simulink model "positionControlSlidingCircle"  (Simulink 7.5)
settings: Solver=FixedStepDiscrete  StartTime=0.0  StopTime=Inf  FixedStep=Ts  RelTol=1e-3
PostLoadFcn:
  | , if any(exist('dsrtsu_mdlpostloadfcn', 'file') == [2, 3, 6]), try dsrtsu_mdlpostloadfcn('Execute', bdroot); catch fprintf('Error in PostLoadFcn (dsrtsu_mdlpostloadfcn) for model "%s":\n %s\n', bdroot, lasterr); end, end,
values from neighbouring files (symbols this model uses):
  bLP = exp(-Wcut*2*pi*Ts)    [main2.m]
  circX = circXt(1:floor(length(circXt)))    [main.m]    (also in main2.m = circX(1:floor(length(circX)/factor)))
  circXd = circXd(1:floor(length(circX)/factor))    [main2.m]
  circXdd = circXdd(1:floor(length(circX)/factor))    [main2.m]
  circY = circYt(1:floor(length(circYt)))    [main.m]    (also in main2.m = circY(1:floor(length(circY)/factor)))
  circYd = circYd(1:floor(length(circY)/factor))    [main2.m]
  circYdd = circYdd(1:floor(length(circY)/factor))    [main2.m]
  cx = 0.001651705312519    (= 0.00165170531252)    [main2.m]
  cy = 0.001046707328795    (= 0.00104670732879)    [main2.m]
  Kd = [5 0;0 5]*10^-4    [main2.m]
  kNorm = 1*10^-1    (= 0.1)    [main2.m]
  Kp = [8 0; 0 7]*10^-2    [main2.m]
  Ks = [7 0;0 0.7]*10^-2    [main2.m]
  Minv = inv(M)    [main2.m]
  mx = 9.241410334340282e-004    (= 0.000924141033434)    [main2.m]
  my = 5.572114462326005e-004    (= 0.000557211446233)    [main2.m]
  r0 = rad    [main2.m]
  rNormal = 109.08    [main2.m]
  Ts = 0.01    [main.m]    (also in main2.m = 0.001)
undefined symbols (not defined in the file or in its folder): DiscIntNeverNeededParam, xc, yc
libraries: rtilib1103 x12, dspinverses x2, dspmtrx3 x2
settings Model: DSRTSU_INTERNAL_RTI_VER=360  DSRTSU_INTERNAL_RTI_TYPE=rti1103  Creator=daq  LastModifiedBy=daq  BufferReuse=off
settings OptimizationCC: BlockReduction=off  OptimizeBlockIOStorage=off  BufferReuse=off  ExpressionFolding=off  LocalBlockOutputs=off
settings HardwareCC: ProdIntDivRoundTo=Zero  ProdEndianess=BigEndian  ProdHWDeviceType=Generic->Custom  TargetIntDivRoundTo=Zero  TargetEndianess=BigEndian  TargetHWDeviceType=Generic->Custom
settings RTWCC: SystemTargetFile=rti1103.tlc  MakeCommand=make_rti  TemplateMakefile=rti1103.tmf  Description=dSPACE DS1103 Hardware Platform  ProcessScript=rti1103_make_rtw_hook
settings STFCustomTargetCC: ParMdlRefBuildCompliant=on  GeneratePreprocessorConditionals=Disable all  SystemTargetFile=rti1103.tlc
settings GRTTargetCC: CompOptLevelCompliant=off  MatFileLogging=off  ExtModeMexFile=noextcomm
settings CustomProperty: DataType=RTWOptions_EnumType_C__dSPACE_matlab_rti1103_tlc_rti1103_1InitialSimState  Value=RUN
settings EnumStrPairs: String=RUN

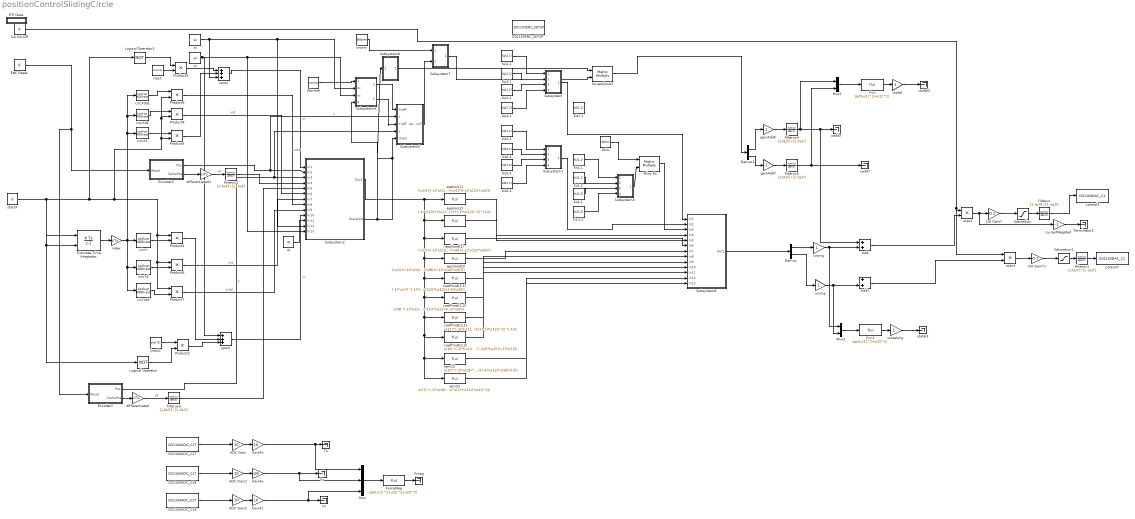
== system positionControlSlidingCircle ==
  " EncoderX" : Subsystem
  " EncoderY" : Subsystem
  -Minv : Constant  Value=-Minv  OutDataType=fixdt(1, 16)  OutScaling=2^0
  -Minv Ks : Product  Multiplication=Matrix(*)  OutDataType=sfix(16)  OutScaling=2^0
  ADC Gain : Gain  Gain=10  ParameterDataType=fixdt(1, 16)  ParameterScaling=2^0  OutDataType=fixdt(1, 16)  OutScaling=2^0
  ADC Gain1 : Gain  Gain=10  ParameterDataType=fixdt(1, 16)  ParameterScaling=2^0  OutDataType=fixdt(1, 16)  OutScaling=2^0
  ADC Gain2 : Gain  Gain=10  ParameterDataType=fixdt(1, 16)  ParameterScaling=2^0  OutDataType=fixdt(1, 16)  OutScaling=2^0
  Add : Sum  OutDataType=fixdt(1, 16)  OutScaling=2^-10
  Add1 : Sum  OutDataType=fixdt(1, 16)  OutScaling=2^-10
  DA GainY : Gain  Gain=0.1  ParameterDataType=fixdt(1, 16)  ParameterScaling=2^0  OutDataType=fixdt(1, 16)  OutScaling=2^0
  DA GainY1 : Gain  Gain=0.1  ParameterDataType=fixdt(1, 16)  ParameterScaling=2^0  OutDataType=fixdt(1, 16)  OutScaling=2^0
  DA On-Off : Constant  Value=0  OutDataType=fixdt(1, 16)  OutScaling=2^0
  DS1103ADC_C17 : rtilib1103/DS1103 MASTER PPC/DS1103ADC_C17  SystemSampleTime=-1  ChannelNo=17  TimerAPreTrigger=0  Reserved2=[]  Reserved3=[]  Reserved4=[]  DialogFcn=gui1103adc  UnitName={ 'DS1103ADC_C' }  UnitValues={ 17 }  DSProperties=struct('RTI',struct('Version',uint32(1),'BlockType',struct('isSLSource',uint8(1),'isSLSink',uint8(0),'isHWSource',uint8(1),'isHWSink',uint8(0),'isSetup',uint8(0),'isInline',uint8(1),'isNonInline',uint8(0),'isInterrupt',uint8(0),'isChannelwise',uint8(1)),'IOBoardType','DS1103MASTER','UnitType','ADC','Identifier','ADC','DialogType','ML','BlockSet','NONE','SlaveProcessor','NONE'))
  DS1103ADC_C18 : rtilib1103/DS1103 MASTER PPC/DS1103ADC_C17  SystemSampleTime=-1  ChannelNo=18  TimerAPreTrigger=0  Reserved2=[]  Reserved3=[]  Reserved4=[]  DialogFcn=gui1103adc  UnitName={ 'DS1103ADC_C' }  UnitValues={ 18 }  DSProperties=struct('RTI',struct('Version',uint32(1),'BlockType',struct('isSLSource',uint8(1),'isSLSink',uint8(0),'isHWSource',uint8(1),'isHWSink',uint8(0),'isSetup',uint8(0),'isInline',uint8(1),'isNonInline',uint8(0),'isInterrupt',uint8(0),'isChannelwise',uint8(1)),'IOBoardType','DS1103MASTER','UnitType','ADC','Identifier','ADC','DialogType','ML','BlockSet','NONE','SlaveProcessor','NONE'))
  DS1103ADC_C19 : rtilib1103/DS1103 MASTER PPC/DS1103ADC_C17  SystemSampleTime=-1  ChannelNo=19  TimerAPreTrigger=0  Reserved2=[]  Reserved3=[]  Reserved4=[]  DialogFcn=gui1103adc  UnitName={ 'DS1103ADC_C' }  UnitValues={ 19 }  DSProperties=struct('RTI',struct('Version',uint32(1),'BlockType',struct('isSLSource',uint8(1),'isSLSink',uint8(0),'isHWSource',uint8(1),'isHWSink',uint8(0),'isSetup',uint8(0),'isInline',uint8(1),'isNonInline',uint8(0),'isInterrupt',uint8(0),'isChannelwise',uint8(1)),'IOBoardType','DS1103MASTER','UnitType','ADC','Identifier','ADC','DialogType','ML','BlockSet','NONE','SlaveProcessor','NONE'))
  DS1103ENC_SETUP : rtilib1103/DS1103 MASTER PPC/DS1103ENC_SETUP  SystemSampleTime=-1  EncRange=0  Reserved1=[]  Reserved2=[]  Reserved3=[]  Reserved4=[]  DialogFcn=gui1103enc_setup  UnitName={ 'DS1103ENC_SETUP' }  UnitValues={ [] }  DSProperties=struct('RTI',struct('Version',uint32(1),'BlockType',struct('isSLSource',uint8(0),'isSLSink',uint8(0),'isHWSource',uint8(0),'isHWSink',uint8(0),'isSetup',uint8(0),'isInline',uint8(1),'isNonInline',uint8(0),'isInterrupt',uint8(0),'isChannelwise',uint8(0)),'IOBoardType','DS1103MASTER','UnitType','ENC','Identifier','ENCMASTER','DialogType','ML','BlockSet','NONE','SlaveProcessor','NONE'))
      settings: SignalType=[0 0 0 0 0 0 0]
  Demux : Demux  Outputs=2
  Demux1 : Demux  Outputs=2
  Discrete-Time Integrator : DiscreteIntegrator  ExternalReset=rising  SampleTime=Ts  OutDataType=fixdt(1, 16)  OutScaling=2^0  ICPrevOutput=DiscIntNeverNeededParam  ICPrevScaledInput=DiscIntNeverNeededParam
  ENC Reset : Constant  Value=0  OutDataType=fixdt(1, 16)  OutScaling=2^0
  Fcn : Fcn  Expr=sqrt(u(1)^2+u(2)^2)
  Fcn1 : Fcn  Expr=sqrt(u(1)^2+u(2)^2)
  Fmag : Terminator
  ForceMag : Fcn  Expr=sqrt(u(1)^2+u(2)^2+u(3)^2)
  Fx : Terminator
  Fy : Terminator
  Fz : Terminator
  GainFx : Gain  Gain=10  ParameterDataType=fixdt(1, 16)  ParameterScaling=2^0  OutDataType=fixdt(1, 16)  OutScaling=2^0
  GainFy : Gain  Gain=100  ParameterDataType=fixdt(1, 16)  ParameterScaling=2^0  OutDataType=fixdt(1, 16)  OutScaling=2^0
  GainFz : Gain  Gain=10  ParameterDataType=fixdt(1, 16)  ParameterScaling=2^0  OutDataType=fixdt(1, 16)  OutScaling=2^0
  Kd1,1 : Constant  Value=Kd(1,1)  OutDataType=fixdt(1, 16)  OutScaling=2^0
  Kd1,3 : Constant  Value=Kd(1,1)  OutDataType=fixdt(1, 16)  OutScaling=2^0
  Kd1,4 : Constant  Value=Kd(1,2)  OutDataType=fixdt(1, 16)  OutScaling=2^0
  Kd2,3 : Constant  Value=Kd(2,1)  OutDataType=fixdt(1, 16)  OutScaling=2^0
  Kd2,4 : Constant  Value=Kd(2,2)  OutDataType=fixdt(1, 16)  OutScaling=2^0
  Kp epsilond1 : Product  Multiplication=Matrix(*)  OutDataType=sfix(16)  OutScaling=2^0
  Kp1,1 : Constant  Value=Kp(1,1)  OutDataType=fixdt(1, 16)  OutScaling=2^0
  Kp1,2 : Constant  Value=Kp(1,2)  OutDataType=fixdt(1, 16)  OutScaling=2^0
  Kp2,1 : Constant  Value=Kp(2,1)  OutDataType=fixdt(1, 16)  OutScaling=2^0
  Kp2,2 : Constant  Value=Kp(2,2)  OutDataType=fixdt(1, 16)  OutScaling=2^0
  Ks 2,2 : Constant  Value=Ks(2,2)  OutDataType=fixdt(1, 16)  OutScaling=2^0
  Ks1,1 : Constant  Value=Ks(1,1)  OutDataType=fixdt(1, 16)  OutScaling=2^0
  Ks1,2 : Constant  Value=Ks(2,1)  OutDataType=fixdt(1, 16)  OutScaling=2^0
  Ks2,1 : Constant  Value=Ks(1,2)  OutDataType=fixdt(1, 16)  OutScaling=2^0
  Logical Operator : Logic  Operator=NOT  AllPortsSameDT=off  OutDataTypeMode=boolean  LogicDataType=fixdt(0, 8)  OutDataTypeStr=boolean
  Logical Operator1 : Logic  Operator=NOT  AllPortsSameDT=off  OutDataTypeMode=boolean  LogicDataType=fixdt(0, 8)  OutDataTypeStr=boolean
  Mux : Mux  Inputs=3
  Mux1 : Mux  Inputs=2
  Mux2 : Mux  Inputs=2
  Product{2..9} (8 alike) : Product  OutDataType=fixdt(1, 16)  OutScaling=2^0  RndMeth=Zero
  RTI Data : Subsystem  Tag=struct('RTIDataServer',struct('RTIDataServerVs','2','RTIModelDescription','struct(''main'',''positionControlSlidingCircle'',''sub'','''',''isMp'',0)'))  LoadFcn="if exist('rtidc'), try,  rtidc('DataHostBlockClbLoad', gcbh); catch, disp(['Warning: ''LoadFcn'' for RTI Data block failed: ' lasterr]); end, end,"
      settings: CopyFcn="if exist('rtidc'), try,  rtidc('DataHostBlockClbCopy', gcbh); catch, disp(['Warning: ''CopyFcn'' for RTI Data block failed: ' lasterr]); end, end,"  DeleteFcn="if exist('rtidc'), try,  rtidc('DataHostBlockClbDelete', gcbh); catch, disp(['Warning: ''DeleteFcn'' for RTI Data block failed: ' lasterr]); end, end,"  ModelCloseFcn="if exist('rtidc'), try,  rtidc('DataHostBlockClbModelClose', gcbh); catch, disp(['Warning: ''ModelCloseFcn'' for RTI Data block failed: ' lasterr]); end, end,"  PreSaveFcn="if exist('rtidc'), try,  rtidc('DataHostBlockClbPreSave', gcbh); catch, disp(['Warning: ''PreSaveFcn'' for RTI Data block failed: ' lasterr]); end, end,"  PostSaveFcn="if exist('rtidc'), try,  rtidc('DataHostBlockClbPostSave', gcbh); catch, disp(['Warning: ''PostSaveFcn'' for RTI Data block failed: ' lasterr]); end, end,"  NameChangeFcn="if exist('rtidc'), try,  rtidc('DataHostBlockClbNameChange', gcbh); catch, disp(['Warning: ''NameChangeFcn'' for RTI Data block failed: ' lasterr]); end, end,"
      mask Type: RTI_DATA_HOST
      mask Description:
      | RTI Data Block.
      | This block is used by RTI to store internal model-dependent data.
      | Please keep this block on the root level of the model. Deleting this block will result in data loss.
      | 
      | NEVER DELETE OR COPY THIS BLOCK!
      mask Help:
      | RTI Data Block.
      | This block is used by RTI to store internal model-dependent data.
      | Please keep this block on the root level of the model. Deleting this block will result in data loss.
      | 
      | NEVER DELETE OR COPY THIS BLOCK!
      mask Display:
      | text(0.5, 0.5, 'RTI Data', 'HorizontalAlignment', 'center');
      | plot([1 0]);
  Saturation : Saturate  UpperLimit=7  LowerLimit=-7  OutDataType=fixdt(1, 16)  OutScaling=2^0
  Saturation1 : Saturate  UpperLimit=7  LowerLimit=-7  OutDataType=fixdt(1, 16)  OutScaling=2^0
  Subsystem : Subsystem
  Subsystem1 : Subsystem
  Subsystem2 : Subsystem
  Subsystem3 : Subsystem
  Subsystem4 : Subsystem
  Subsystem5 : Subsystem
  Subsystem6 : Subsystem
  Subsystem7 : Subsystem
  Subsystem8 : Subsystem
  Terminator1 : Terminator
  circX1 : LookupNDDirect  NumberOfTableDimensions=1  Table=circX
  circXd1 : LookupNDDirect  NumberOfTableDimensions=1  Table=circXd
  circXdd1 : LookupNDDirect  NumberOfTableDimensions=1  Table=circXdd
  circY : LookupNDDirect  NumberOfTableDimensions=1  Table=circY
  circYd : LookupNDDirect  NumberOfTableDimensions=1  Table=circYd
  circYdd : LookupNDDirect  NumberOfTableDimensions=1  Table=circYdd
  coeffmat(1,1) : Fcn  Expr=(-1)*u(17)^(-1)*((u(1)+(-1)*u(11))^2+(u(2)+(-1)*u(12))^2)^(-3/2)*(u(2)+(-1)*u(12))*((-1)*u(11)^2+u(1)*(u(11)+(-1)*u(5))+u(11)*u(5)+(u(2)+(-1)*u(12))*(u(12)+(-1)*u(6)))
  coeffmat(1,2) : Fcn  Expr=u(18)^(-1)*(u(1)+(-1)*u(11))*((u(1)+(-1)*u(11))^2+(u(2)+(-1)*u(12))^2)^(-3/2)*((-1)*u(11)^2+u(1)*(u(11)+(-1)*u(5))+u(11)*u(5)+(u(2)+(-1)*u(12))*(u(12)+(-1)*u(6)))
  coeffmat(2,1) : Fcn  Expr=u(17)^(-1)*(u(1)+(-1)*u(11))*((u(1)+(-1)*u(11))^2+(u(2)+(-1)*u(12))^2)^(-1/2)
  coeffmat(2,2) : Fcn  Expr=u(18)^(-1)*((u(1)+(-1)*u(11))^2+(u(2)+(-1)*u(12))^2)^(-1/2)*(u(2)+(-1)*u(12))
  controlX : rtilib1103/DS1103 MASTER PPC/DS1103DAC_C1  SystemSampleTime=-1  ChannelNo=1  InitValue=0  TermMode=0  TermValue=0  Reserved1=[]  Reserved2=[]  Reserved3=[]  Reserved4=[]  DialogFcn=gui1103dac  UnitName={ 'DS1103DAC_C' }  UnitValues={ 1 }  DSProperties=struct('RTI',struct('Version',uint32(1),'BlockType',struct('isSLSource',uint8(0),'isSLSink',uint8(1),'isHWSource',uint8(0),'isHWSink',uint8(1),'isSetup',uint8(0),'isInline',uint8(1),'isNonInline',uint8(0),'isInterrupt',uint8(0),'isChannelwise',uint8(1)),'IOBoardType','DS1103MASTER','UnitType','DAC','Identifier','DAC','DialogType','ML','BlockSet','NONE','SlaveProcessor','NONE'))
  controlY : rtilib1103/DS1103 MASTER PPC/DS1103DAC_C1  SystemSampleTime=-1  ChannelNo=2  InitValue=0  TermMode=1  TermValue=0  Reserved1=[]  Reserved2=[]  Reserved3=[]  Reserved4=[]  DialogFcn=gui1103dac  UnitName={ 'DS1103DAC_C' }  UnitValues={ 2 }  DSProperties=struct('RTI',struct('Version',uint32(1),'BlockType',struct('isSLSource',uint8(0),'isSLSink',uint8(1),'isHWSource',uint8(0),'isHWSink',uint8(1),'isSetup',uint8(0),'isInline',uint8(1),'isNonInline',uint8(0),'isInterrupt',uint8(0),'isChannelwise',uint8(1)),'IOBoardType','DS1103MASTER','UnitType','DAC','Identifier','DAC','DialogType','ML','BlockSet','NONE','SlaveProcessor','NONE'))
  currentNegated : Gain  Gain=-1  ParameterDataType=fixdt(1, 16)  ParameterScaling=2^0  OutDataType=fixdt(1, 16)  OutScaling=2^0
  differentiated : Gain  Gain=1/Ts  ParameterDataType=fixdt(1, 16)  ParameterScaling=2^0  OutDataType=fixdt(1, 16)  OutScaling=2^0
  differentiated1 : Gain  Gain=1/Ts  ParameterDataType=fixdt(1, 16)  ParameterScaling=2^0  OutDataType=fixdt(1, 16)  OutScaling=2^0
  epsilon(1) : Fcn  Expr=((u(1)+(-1)*u(11))^2+(u(2)+(-1)*u(12))^2)^(-1/2)*(u(5)*((-1)*u(2)+u(12))+u(11)*(u(2)+(-1)*u(6))+u(1)*((-1)*u(12)+u(6)))
  epsilon(2) : Fcn  Expr=(-1)*u(13)+((u(1)+(-1)*u(11))^2+(u(2)+(-1)*u(12))^2)^(1/2)
  epsilond(1) : Fcn  Expr=((u(1)+(-1)*u(11))^2+(u(2)+(-1)*u(12))^2)^(-3/2)*(u(11)^2*(u(3)*u(2)+(-1)*u(7)*u(2)+(-1)*u(3)*u(12)+u(7)*u(12)+(-1)*u(5)*u(4))+(-1)*(u(2)+(-1)*u(12))^2*(u(7)*u(2)+u(3)*u(12)+(-1)*u(7)*u(12)+(-1)*u(3)*u(6))+u(11)^3*(u(4)+(-1)*u(8))+u(1)^3*u(8)+u(1)^2*(u(7)*((-1)*u(2)+u(12))+u(11)*u(4)+(-1)*u(5)*u(4)+(-3)*u(11)*u(8))+(-1)*u(11)*(u(2)+(-1)*u(12))*(u(3)*u(5)+u(12)*u(4)+(-1)*u(4)*u(6)+u(2)*u(8)+(-1)*u(12)*u(8))+u(1)*(u(11)*((-1)*u(3)*u(2)+2*u(7)*u(2)+u(3)*u(12)+(-2)*u(7)*u(12)+2*u(5)*u(4))+u(11)^2*((-2)*u(4)+3*u(8))+(u(2)+(-1)*u(12))*(u(3)*u(5)+u(12)*u(4)+(-1)*u(4)*u(6)+u(2)*u(8)+(-1)*u(12)*u(8))))
  epsilond(2) : Fcn  Expr=((u(1)+(-1)*u(11))^2+(u(2)+(-1)*u(12))^2)^(-3/2)*(u(11)^2*(u(3)*u(2)+(-1)*u(7)*u(2)+(-1)*u(3)*u(12)+u(7)*u(12)+(-1)*u(5)*u(4))+(-1)*(u(2)+(-1)*u(12))^2*(u(7)*u(2)+u(3)*u(12)+(-1)*u(7)*u(12)+(-1)*u(3)*u(6))+u(11)^3*(u(4)+(-1)*u(8))+u(1)^3*u(8)+u(1)^2*(u(7)* ((-1)*u(2)+u(12))+u(11)*u(4)+(-1)*u(5)*u(4)+(-3)*u(11)*u(8))+(-1)*u(11)*(u(2)+(-1)*u(12))*(u(3)*u(5)+u(12)*u(4)+(-1)*u(4)*u(6)+u(2)*u(8)+(-1)*u(12)*u(8))+u(1)*(u(11)*((-1)*u(3)*u(2)+2*u(7)*u(2)+u(3)*u(12)+(-2)*u(7)*u(12)+2*u(5)*u(4))+u(11)^2*((-2)*u(4)+3*u(8))+(u(2)+(-1)*u(12))*(u(3)*u(5)+u(12)*u(4)+(-1)*u(4)*u(6)+u(2)*u(8)+(-1)*u(12)*u(8))))
  filterux{,1..5} (6 alike) : DiscreteFilter  Numerator=[1-bLP]  Denominator=[1 -bLP]
  gainAddX : Gain  ParameterDataType=fixdt(1, 16)  ParameterScaling=2^0  OutDataType=fixdt(1, 16)  OutScaling=2^0
  gainAddY : Gain  ParameterDataType=fixdt(1, 16)  ParameterScaling=2^0  OutDataType=fixdt(1, 16)  OutScaling=2^0
  index : Gain  Gain=1/Ts  ParameterDataType=fixdt(1, 16)  ParameterScaling=2^0  OutDataType=fixdt(1, 16)  OutScaling=2^0
  input : Constant  Value=circX(1)  OutDataType=fixdt(1, 16)  OutScaling=2^0
  input2 : Constant  Value=circY(1)  OutDataType=fixdt(1, 16)  OutScaling=2^0
  knorm : Constant  Value=kNorm  OutDataType=fixdt(1, 16)  OutScaling=2^0
  r0 : Constant  Value=r0  OutDataType=fixdt(1, 16)  OutScaling=2^0
  rNormal : Constant  Value=rNormal  OutDataType=fixdt(1, 16)  OutScaling=2^0
  rem(1) : Fcn  Expr=u(17)^(-1)*u(18)^(-1)*((u(1)+(-1)*u(11))^2+(u(2)+(-1)*u(12))^2)^(-5/2)*(u(15)*u(18)*u(3)*(u(1)^2+(-2)*u(1)*u(11)+u(11)^2+(u(2)+(-1)*u(12))^2)*(u(2)+(-1)*u(12))*((-1)*u(11)^2+u(1)*(u(11)+(-1)*u(5))+u(11)*u(5)+(u(2)+(-1)*u(12))*(u(12)+(-1)*u(6)))+u(17)*((-1)*u(16)*(u(1)+(-1)*u(11))*(u(1)^2+(-2)*u(1)*u(11)+u(11)^2+(u(2)+(-1)*u(12))^2)*u(4)*((-1)*u(11)^2+u(1)*(u(11)+(-1)*u(5))+u(11)*u(5)+(u(2)+(-1)*u(12))*(u(12)+(-1)*u(6)))+u(18)*(u(11)^4*(u(9)*((-1)*u(2)+u(12))+2*(u(3)+(-1)*u(7))*u(4))+(u(2)+(-1)*u(12))^3*(u(3)^2*u(5)+(-1)*u(9)*(u(2)+(-1)*u(12))^2+2*u(3)*((-1)*u(4)*u(6)+u(12)*(u(4)+(-1)*u(8))+u(2)*u(8)))+(-1)*u(11)^2*(u(2)+(-1)*u(12))*(2*u(3)^2*u(5)+2*u(9)*(u(2)+(-1)*u(12))^2+u(4)*(2*u(7)*u(2)+(-2)*u(7)*u(12)+(-3)*u(5)*u(4))+2*u(3)*(2*u(2)*u(4)+(-2)*u(4)*u(6)+(-1)*u(2)*u(8)+u(12)*u(8)))+u(1)^5*u(10)+(-1)*u(11)^5*u(10)+(-1)*u(1)^4*(u(9)*(u(2)+(-1)*u(12))+2*u(7)*u(4)+5*u(11)*u(10))+u(1)^3*(u(12)*u(4)^2+2*u(3)*(u(7)*(u(2)+(-1)*u(12))+((-1)*u(11)+u(5))*u(4))+4*u(11)*(u(9)*u(2)+(-1)*u(9)*u(12)+2*u(7)*u(4))+(-1)*u(4)^2*u(6)+(-2)*u(2)*u(4)*u(8)+2*u(12)*u(4)*u(8)+10*u(11)^2*u(10)+2*u(2)^2*u(10)+(-4)*u(2)*u(12)*u(10)+2*u(12)^2*u(10))+(-1)*u(11)*(u(2)+(-1)*u(12))^2*(2*u(3)*(u(7)*(u(2)+(-1)*u(12))+(-2)*u(5)*u(4))+u(3)^2*(u(2)+2*u(12)+(-3)*u(6))+2*u(4)^2*u(6)+(-2)*u(2)*u(4)*u(8)+u(2)^2*u(10)+u(12)^2*u(10)+(-2)*u(12)*(u(4)^2+(-1)*u(4)*u(8)+u(2)*u(10)))+u(11)^3*(2*u(3)^2*(u(2)+(-1)*u(12))+2*u(12)*u(4)^2+(-2)*u(3)*(u(7)*(u(2)+(-1)*u(12))+u(5)*u(4))+u(4)^2*u(6)+(-2)*u(12)*u(4)*u(8)+(-2)*u(2)^2*u(10)+(-2)*u(12)^2*u(10)+u(2)*((-3)*u(4)^2+2*u(4)*u(8)+4*u(12)*u(10)))+u(1)*(u(11)^3*(4*u(9)*(u(2)+(-1)*u(12))+(-6)*u(3)*u(4)+8*u(7)*u(4))+2*u(11)*(u(2)+(-1)*u(12))*(2*u(3)^2*u(5)+2*u(9)*(u(2)+(-1)*u(12))^2+u(4)*(2*u(7)*(u(2)+(-1)*u(12))+(-3)*u(5)*u(4))+2*u(3)*((-2)*u(4)*u(6)+u(2)*(u(4)+(-1)*u(8))+u(12)*(u(4)+u(8))))+5*u(11)^4*u(10)+(u(2)+(-1)*u(12))^2*(2*u(3)*(u(7)*(u(2)+(-1)*u(12))+(-2)*u(5)*u(4))+3*u(3)^2*(u(12)+(-1)*u(6))+2*u(4)^2*u(6)+(-2)*u(2)*u(4)*u(8)+u(2)^2*u(10)+u(12)^2*u(10)+(-2)*u(12)*(u(4)^2+(-1)*u(4)*u(8)+u(2)*u(10)))+u(11)^2*((-4)*u(3)^2*(u(2)+(-1)*u(12))+(-3)*u(12)*u(4)^2+6*u(3)*(u(7)*(u(2)+(-1)*u(12))+u(5)*u(4))+(-3)*u(4)^2*u(6)+6*u(12)*u(4)*u(8)+6*u(2)^2*u(10)+6*u(12)^2*u(10)+6*u(2)*(u(4)^2+(-1)*u(4)*u(8)+(-2)*u(12)*u(10))))+(-1)*u(1)^2*(6*u(11)^2*(u(9)*u(2)+(-1)*u(9)*u(12)+(-1)*u(3)*u(4)+2*u(7)*u(4))+(u(2)+(-1)*u(12))*(2*u(3)^2*u(5)+2*u(9)*(u(2)+(-1)*u(12))^2+u(4)*(2*u(7)*u(2)+(-2)*u(7)*u(12)+(-3)*u(5)*u(4))+2*u(3)*((-2)*u(4)*u(6)+(-1)*u(2)*u(8)+u(12)*(2*u(4)+u(8))))+10*u(11)^3*u(10)+u(11)*((-2)*u(3)^2*(u(2)+(-1)*u(12))+6*u(3)*(u(7)*(u(2)+(-1)*u(12))+u(5)*u(4))+3*((-1)*u(4)^2*u(6)+2*u(12)*u(4)*u(8)+2*u(2)^2*u(10)+2*u(12)^2*u(10)+u(2)*(u(4)^2+(-2)*u(4)*u(8)+(-4)*u(12)*u(10))))))))
  rem(2) : Fcn  Expr=u(17)^(-1)*u(18)^(-1)*((u(1)+(-1)*u(11))^2+(u(2)+(-1)*u(12))^2)^(-3/2)*((-1)*u(15)*u(18)*(u(1)+(-1)*u(11))*u(3)*(u(1)^2+(-2)*u(1)*u(11)+u(11)^2+(u(2)+(-1)*u(12))^2)+u(17)*((-1)*u(16)*(u(1)^2+(-2)*u(1)*u(11)+u(11)^2+(u(2)+(-1)*u(12))^2)*(u(2)+(-1)*u(12))*u(4)+u(18)*(u(3)*(u(2)+(-1)*u(12))+((-1)*u(1)+u(11))*u(4))^2))
  startX : Constant  Value=0  OutDataType=fixdt(1, 16)  OutScaling=2^0
  uaddX : Terminator
  uaddY : Terminator
  utotal : Gain  ParameterDataType=fixdt(1, 16)  ParameterScaling=2^0  OutDataType=fixdt(1, 16)  OutScaling=2^0
  utotal2 : Terminator
  utotal3 : Terminator
  utotalorig : Gain  ParameterDataType=fixdt(1, 16)  ParameterScaling=2^0  OutDataType=fixdt(1, 16)  OutScaling=2^0
  uxact : Product  OutDataType=fixdt(1, 16)  OutScaling=2^0  RndMeth=Zero
  uxorig : Gain  ParameterDataType=fixdt(1, 16)  ParameterScaling=2^0  OutDataType=fixdt(1, 16)  OutScaling=2^0
  uyact : Product  OutDataType=fixdt(1, 16)  OutScaling=2^0  RndMeth=Zero
  uyorig : Gain  ParameterDataType=fixdt(1, 16)  ParameterScaling=2^0  OutDataType=fixdt(1, 16)  OutScaling=2^0
  xc : Constant  Value=xc  OutDataType=fixdt(1, 16)  OutScaling=2^0
  xposr : Sum  Inputs=+++  OutDataType=fixdt(1, 16)  OutScaling=2^-10
  yc : Constant  Value=yc  OutDataType=fixdt(1, 16)  OutScaling=2^0
  yposr : Sum  Inputs=+++  OutDataType=fixdt(1, 16)  OutScaling=2^-10
  wires:
  DA GainY/1 -> Saturation/1
  uxact/1 -> DA GainY/1, currentNegated/1
  DA On-Off/1 -> uxact/1, uyact/1
  ENC Reset/1 -> " EncoderX"/1(Reset), " EncoderY"/1(Reset)
  DS1103ADC_C18/1 -> ADC Gain1/1
  GainFz/1 -> Fz/1, Mux/3
  DS1103ADC_C17/1 -> ADC Gain/1
  ADC Gain/1 -> GainFx/1
  ADC Gain1/1 -> GainFy/1
  ADC Gain2/1 -> GainFz/1
  GainFy/1 -> Fy/1, Mux/2
  currentNegated/1 -> Terminator1/1
  " EncoderX"/2(DeltaPos) -> differentiated1/1
  GainFx/1 -> Fx/1, Mux/1
  DS1103ADC_C19/1 -> ADC Gain2/1
  startX/1 -> Discrete-Time Integrator/1, Discrete-Time Integrator/2, Logical Operator/1, Logical Operator1/1, Product4/1, Product6/1, Product7/1, Product5/2, Product8/2, Product9/2
  Discrete-Time Integrator/1 -> index/1
  index/1 -> circY/1, circYd/1, circYdd/1, circX1/1, circXd1/1, circXdd1/1
  differentiated1/1 -> filterux2/1  "xd"
  differentiated/1 -> filterux3/1  "yd"
  uyact/1 -> DA GainY1/1
  input2/1 -> Product2/1
  Logical Operator/1 -> Product2/2
  input/1 -> Product3/2
  Product3/1 -> xposr/1
  Logical Operator1/1 -> Product3/1
  circY/1 -> Product4/2
  circX1/1 -> Product5/1
  Product5/1 -> xposr/2
  circYd/1 -> Product6/2
  circYdd/1 -> Product7/2
  circXd1/1 -> Product8/1
  circXdd1/1 -> Product9/1
  " EncoderX"/1(Pos) -> Subsystem2/2(In2), Subsystem5/2(x)  "x"
  " EncoderY"/1(Pos) -> Subsystem2/3(In3), Subsystem5/4(y)  "y"
  " EncoderY"/2(DeltaPos) -> differentiated/1
  Product8/1 -> Subsystem2/6(In6)  "xrd"
  Product9/1 -> Subsystem2/8(In8)  "xrdd"
  Product6/1 -> Subsystem2/7(In7)  "yrd"
  Product7/1 -> Subsystem2/9(In9)  "yrdd"
  Subsystem2/1(Out1) -> epsilon(1)/1, epsilon(2)/1, epsilond(1)/1, epsilond(2)/1, coeffmat(1,1)/1, coeffmat(1,2)/1, coeffmat(2,1)/1, coeffmat(2,2)/1, rem(1)/1, rem(2)/1
  epsilon(2)/1 -> Subsystem8/5(In5)
  epsilond(1)/1 -> Subsystem8/6(In6)
  epsilond(2)/1 -> Subsystem8/7(In7)
  rem(1)/1 -> Subsystem8/12(In12)
  rem(2)/1 -> Subsystem8/13(In13)
  epsilon(1)/1 -> Subsystem8/4(In4)
  coeffmat(1,1)/1 -> Subsystem8/8(In8)
  coeffmat(1,2)/1 -> Subsystem8/9(In9)
  coeffmat(2,1)/1 -> Subsystem8/10(In10)
  coeffmat(2,2)/1 -> Subsystem8/11(In11)
  Subsystem8/1(Out1) -> Demux/1
  DA GainY1/1 -> Saturation1/1
  Saturation/1 -> filterux/1
  Saturation1/1 -> filterux1/1
  filterux/1 -> controlX/1
  filterux1/1 -> controlY/1
  xposr/1 -> Subsystem2/1(In1)  "xr"
  yposr/1 -> Subsystem2/10(In10)  "yr"
  Mux/1 -> ForceMag/1
  ForceMag/1 -> Fmag/1
  filterux2/1 -> Subsystem2/4(In4)
  filterux3/1 -> Subsystem2/5(In5)
  r0/1 -> Subsystem2/11(In11)
  rNormal/1 -> Subsystem4/1(rnew)
  xc/1 -> xposr/3, Subsystem4/2(xc), Subsystem2/12(In12)
  yc/1 -> yposr/1, Subsystem4/3(yc), Subsystem2/13(In13)
  Subsystem4/1(xrefF) -> Subsystem5/1(XrefF)
  Subsystem4/2(yrefF) -> Subsystem5/3(YrefF)
  knorm/1 -> Subsystem7/1(In1)
  Subsystem5/1(epsilonnF) -> Subsystem7/2(In2)
  Subsystem2/2(thetaOut) -> Subsystem4/4(theta), Subsystem5/5(theta), Subsystem6/1(In1)
  Subsystem6/1(Out1) -> Kp epsilond1/1
  Subsystem7/1(Out1) -> Kp epsilond1/2
  Kp epsilond1/1 -> Demux1/1
  Demux1/1 -> gainAddX/1
  Demux1/2 -> gainAddY/1
  Subsystem3/1(Out1) -> -Minv Ks/2
  Ks 2,2/1 -> Subsystem3/4(In4)
  Ks2,1/1 -> Subsystem3/3(In3)
  Ks1,2/1 -> Subsystem3/2(In2)
  Ks1,1/1 -> Subsystem3/1(In1)
  Kd2,4/1 -> Subsystem1/4(In4)
  Kd1,4/1 -> Subsystem1/3(In3)
  Kd2,3/1 -> Subsystem1/2(In2)
  Kd1,3/1 -> Subsystem1/1(In1)
  Kp2,2/1 -> Subsystem/4(In4)
  Kp1,2/1 -> Subsystem/3(In3)
  Kp2,1/1 -> Subsystem/2(In2)
  Kp1,1/1 -> Subsystem/1(In1)
  -Minv Ks/1 -> Subsystem8/3(In3)
  -Minv/1 -> -Minv Ks/1
  Subsystem/1(Out1) -> Subsystem8/1(In1)
  Subsystem1/1(Out1) -> Subsystem8/2(In2)
  gainAddX/1 -> filterux4/1
  Demux/1 -> uxorig/1
  Add/1 -> uxact/2
  Demux/2 -> uyorig/1
  Add1/1 -> uyact/2
  uxorig/1 -> Add/2, Mux2/1
  uyorig/1 -> Add1/2, Mux2/2
  Mux1/1 -> Fcn/1
  Fcn/1 -> utotal/1
  utotal/1 -> utotal2/1
  filterux4/1 -> uaddX/1, Add/1, Mux1/1
  Product2/1 -> yposr/3
  Product4/1 -> yposr/2
  gainAddY/1 -> filterux5/1
  filterux5/1 -> uaddY/1, Mux1/2
  Mux2/1 -> Fcn1/1
  Fcn1/1 -> utotalorig/1
  utotalorig/1 -> utotal3/1

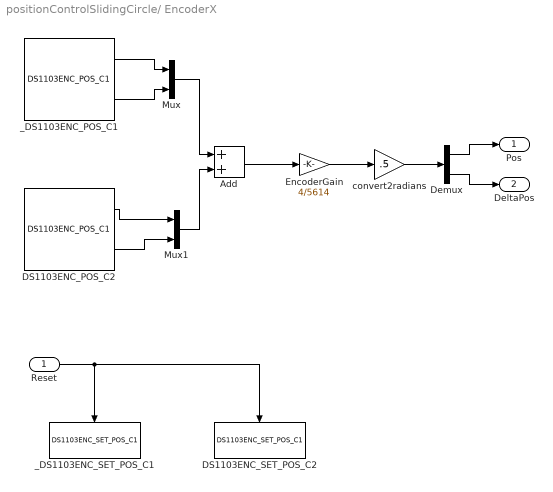
== system positionControlSlidingCircle/ EncoderX ==
  Reset : Inport
  Add : Sum  OutDataType=fixdt(1, 16)  OutScaling=2^-10
  DS1103ENC_POS_C2 : rtilib1103/DS1103 MASTER PPC/DS1103ENC_POS_C1  SystemSampleTime=-1  ChannelNo=2  PosValue=0  Reserved1=[]  Reserved2=[]  Reserved3=[]  Reserved4=[]  DialogFcn=gui1103enc_pos  UnitName={ 'DS1103ENC_POS_C' }  UnitValues={ 2 }  DSProperties=struct('RTI',struct('Version',uint32(1),'BlockType',struct('isSLSource',uint8(1),'isSLSink',uint8(0),'isHWSource',uint8(1),'isHWSink',uint8(0),'isSetup',uint8(0),'isInline',uint8(1),'isNonInline',uint8(0),'isInterrupt',uint8(0),'isChannelwise',uint8(1)),'IOBoardType','DS1103MASTER','UnitType','ENC','Identifier','ENCPOSCH','DialogType','ML','BlockSet','NONE','SlaveProcessor','NONE'))
  DS1103ENC_SET_POS_C2 : rtilib1103/DS1103 MASTER PPC/DS1103ENC_SET_POS_C1  SystemSampleTime=-1  ChannelNo=2  PosValue=0  Reserved1=[]  Reserved2=[]  Reserved3=[]  Reserved4=[]  DialogFcn=gui1103enc_set_pos  UnitName={ 'DS1103ENC_SET_POS_C' }  UnitValues={ 2 }  DSProperties=struct('RTI',struct('Version',uint32(1),'BlockType',struct('isSLSource',uint8(0),'isSLSink',uint8(1),'isHWSource',uint8(0),'isHWSink',uint8(1),'isSetup',uint8(0),'isInline',uint8(1),'isNonInline',uint8(0),'isInterrupt',uint8(0),'isChannelwise',uint8(1)),'IOBoardType','DS1103MASTER','UnitType','ENC','Identifier','ENCRESET','DialogType','ML','BlockSet','NONE','SlaveProcessor','NONE'))
  Demux : Demux  Outputs=2
  EncoderGain : Gain  Gain=4/5614  SaturateOnIntegerOverflow=on  OutDataTypeStr=Inherit: Same as input  ParamDataTypeStr=Inherit: Same as input
  Mux : Mux  Inputs=2
  Mux1 : Mux  Inputs=2
  _DS1103ENC_POS_C1 : rtilib1103/DS1103 MASTER PPC/DS1103ENC_POS_C1  SystemSampleTime=-1  ChannelNo=1  PosValue=0  Reserved1=[]  Reserved2=[]  Reserved3=[]  Reserved4=[]  DialogFcn=gui1103enc_pos  UnitName={ 'DS1103ENC_POS_C' }  UnitValues={ 1 }  DSProperties=struct('RTI',struct('Version',uint32(1),'BlockType',struct('isSLSource',uint8(1),'isSLSink',uint8(0),'isHWSource',uint8(1),'isHWSink',uint8(0),'isSetup',uint8(0),'isInline',uint8(1),'isNonInline',uint8(0),'isInterrupt',uint8(0),'isChannelwise',uint8(1)),'IOBoardType','DS1103MASTER','UnitType','ENC','Identifier','ENCPOSCH','DialogType','ML','BlockSet','NONE','SlaveProcessor','NONE'))
  _DS1103ENC_SET_POS_C1 : rtilib1103/DS1103 MASTER PPC/DS1103ENC_SET_POS_C1  SystemSampleTime=-1  ChannelNo=1  PosValue=0  Reserved1=[]  Reserved2=[]  Reserved3=[]  Reserved4=[]  DialogFcn=gui1103enc_set_pos  UnitName={ 'DS1103ENC_SET_POS_C' }  UnitValues={ 1 }  DSProperties=struct('RTI',struct('Version',uint32(1),'BlockType',struct('isSLSource',uint8(0),'isSLSink',uint8(1),'isHWSource',uint8(0),'isHWSink',uint8(1),'isSetup',uint8(0),'isInline',uint8(1),'isNonInline',uint8(0),'isInterrupt',uint8(0),'isChannelwise',uint8(1)),'IOBoardType','DS1103MASTER','UnitType','ENC','Identifier','ENCRESET','DialogType','ML','BlockSet','NONE','SlaveProcessor','NONE'))
  "convert2radians " : Gain  Gain=.5
  Pos : Outport
  DeltaPos : Outport  Port=2
  wires:
  _DS1103ENC_POS_C1/1 -> Mux/1
  _DS1103ENC_POS_C1/2 -> Mux/2
  EncoderGain/1 -> "convert2radians "/1
  "convert2radians "/1 -> Demux/1
  Reset/1 -> _DS1103ENC_SET_POS_C1/Trigger, DS1103ENC_SET_POS_C2/Trigger
  Mux/1 -> Add/1
  Demux/1 -> Pos/1
  Demux/2 -> DeltaPos/1
  Mux1/1 -> Add/2
  DS1103ENC_POS_C2/1 -> Mux1/1
  DS1103ENC_POS_C2/2 -> Mux1/2
  Add/1 -> EncoderGain/1

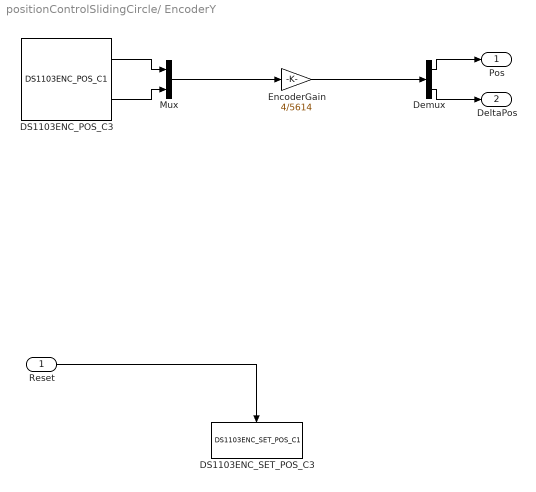
== system positionControlSlidingCircle/ EncoderY ==
  Reset : Inport
  DS1103ENC_POS_C3 : rtilib1103/DS1103 MASTER PPC/DS1103ENC_POS_C1  SystemSampleTime=-1  ChannelNo=3  PosValue=0  Reserved1=[]  Reserved2=[]  Reserved3=[]  Reserved4=[]  DialogFcn=gui1103enc_pos  UnitName={ 'DS1103ENC_POS_C' }  UnitValues={ 3 }  DSProperties=struct('RTI',struct('Version',uint32(1),'BlockType',struct('isSLSource',uint8(1),'isSLSink',uint8(0),'isHWSource',uint8(1),'isHWSink',uint8(0),'isSetup',uint8(0),'isInline',uint8(1),'isNonInline',uint8(0),'isInterrupt',uint8(0),'isChannelwise',uint8(1)),'IOBoardType','DS1103MASTER','UnitType','ENC','Identifier','ENCPOSCH','DialogType','ML','BlockSet','NONE','SlaveProcessor','NONE'))
  DS1103ENC_SET_POS_C3 : rtilib1103/DS1103 MASTER PPC/DS1103ENC_SET_POS_C1  SystemSampleTime=-1  ChannelNo=3  PosValue=0  Reserved1=[]  Reserved2=[]  Reserved3=[]  Reserved4=[]  DialogFcn=gui1103enc_set_pos  UnitName={ 'DS1103ENC_SET_POS_C' }  UnitValues={ 3 }  DSProperties=struct('RTI',struct('Version',uint32(1),'BlockType',struct('isSLSource',uint8(0),'isSLSink',uint8(1),'isHWSource',uint8(0),'isHWSink',uint8(1),'isSetup',uint8(0),'isInline',uint8(1),'isNonInline',uint8(0),'isInterrupt',uint8(0),'isChannelwise',uint8(1)),'IOBoardType','DS1103MASTER','UnitType','ENC','Identifier','ENCRESET','DialogType','ML','BlockSet','NONE','SlaveProcessor','NONE'))
  Demux : Demux  Outputs=2
  EncoderGain : Gain  Gain=4/5614  SaturateOnIntegerOverflow=on  OutDataTypeStr=Inherit: Same as input  ParamDataTypeStr=Inherit: Same as input
  Mux : Mux  Inputs=2
  Pos : Outport
  DeltaPos : Outport  Port=2
  wires:
  Mux/1 -> EncoderGain/1
  Demux/2 -> DeltaPos/1
  Demux/1 -> Pos/1
  Reset/1 -> DS1103ENC_SET_POS_C3/Trigger
  EncoderGain/1 -> Demux/1
  DS1103ENC_POS_C3/2 -> Mux/2
  DS1103ENC_POS_C3/1 -> Mux/1

== system positionControlSlidingCircle/RTI Data ==
  RTI Data Store : Subsystem  Tag="struct('private',struct('version',struct('dsVer',uint32(2),'dsVerCreation',uint32(2),'RTI',struct('ver','6.5','type','RTI1103')),'access',struct('type','Model','isPerm',1,'created',['16-Oct-2016 18:11:40'],'modified',['05-May-2017 14:24:47'],'location','')),'public',struct('main',struct('data',[]),'sub',struct('name',{{'positionControlSlidingCircle'}},'data',{{struct('TH',struct('thTaskInfo',struct('taskType',{'TIMER','HWINT','TMRINT','SWINT'},'tasksNumOf',{1,0,0,0},'srcIds',{{'TIMERA'},{},{},{}},'taskNames',{{['Timer Task 1']},{},{},{}})),'th_tc',struct('dataType','TASK','taskGroupId','','taskGroupList',{{}},'taskSchedulingPolicy','FCFS','taskType','TIMER','blkh',-1,'srcId','TIMERA','srcSgnName',['Timer A interrupt'],'srcCpuName','','taskName',['Timer Task 1  [0.001] s'],'taskNameDisplayExt','','smplTime',0.001,'smplTimeOffs',0,'hasFixedPriority',0,'priority',1,'hasFixedOvc',0,'ovcType',1,'ovcMax',1),'tc_th',struct('dataType','TASK','taskGroupId','','taskGroupList',{{}},'taskSchedulingPolicy','FCFS','taskType','TIMER','blkh',-1,'srcId','TIMERA','srcSgnName',['Timer A interrupt'],'srcCpuName','','taskName',['Timer Task 1  [0.001] s'],'taskNameDisplayExt','','smplTime',0.001,'smplTimeOffs',0,'hasFixedPriority',0,'priority',1,'hasFixedOvc',0,'ovcType',1,'ovcMax',1))}})))"
      mask Type: RTI_DATA_STORE
      mask Description:
      | RTI Data Store Block. This block is used by RTI to store internal model dependent data. Deleting this block will result in data loss.
      | 
      | NEVER DELETE, COPY, OR MODIFY THIS BLOCK!
      mask Help:
      | RTI Data Store Block. This block is used by RTI to store internal model dependent data. Deleting this block will result in data loss.
      | 
      | NEVER DELETE, COPY, OR MODIFY THIS BLOCK!
      mask Display: text(0.5, 0.5, ' ', 'HorizontalAlignment', 'center');

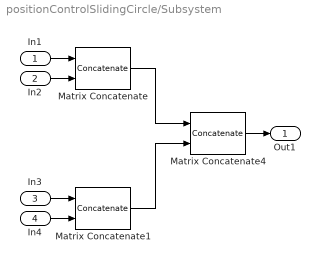
== system positionControlSlidingCircle/Subsystem ==
  In1 : Inport
  In2 : Inport  Port=2
  In3 : Inport  Port=3
  In4 : Inport  Port=4
  Matrix Concatenate : Concatenate  Mode=Vector  ConcatenateDimension=2
  Matrix Concatenate1 : Concatenate  Mode=Vector  ConcatenateDimension=2
  Matrix Concatenate4 : Concatenate  Mode=Multidimensional array  ConcatenateDimension=2
  Out1 : Outport
  wires:
  Matrix Concatenate/1 -> Matrix Concatenate4/1
  Matrix Concatenate1/1 -> Matrix Concatenate4/2
  In1/1 -> Matrix Concatenate/1
  In2/1 -> Matrix Concatenate/2
  Matrix Concatenate4/1 -> Out1/1
  In3/1 -> Matrix Concatenate1/1
  In4/1 -> Matrix Concatenate1/2

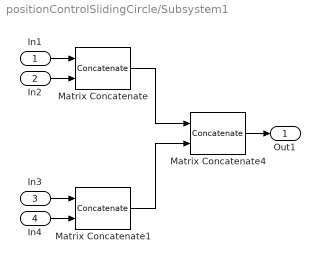
== system positionControlSlidingCircle/Subsystem1 ==
  In1 : Inport
  In2 : Inport  Port=2
  In3 : Inport  Port=3
  In4 : Inport  Port=4
  Matrix Concatenate : Concatenate  Mode=Vector  ConcatenateDimension=2
  Matrix Concatenate1 : Concatenate  Mode=Vector  ConcatenateDimension=2
  Matrix Concatenate4 : Concatenate  Mode=Multidimensional array  ConcatenateDimension=2
  Out1 : Outport
  wires:
  Matrix Concatenate/1 -> Matrix Concatenate4/1
  Matrix Concatenate1/1 -> Matrix Concatenate4/2
  In1/1 -> Matrix Concatenate/1
  In2/1 -> Matrix Concatenate/2
  Matrix Concatenate4/1 -> Out1/1
  In3/1 -> Matrix Concatenate1/1
  In4/1 -> Matrix Concatenate1/2

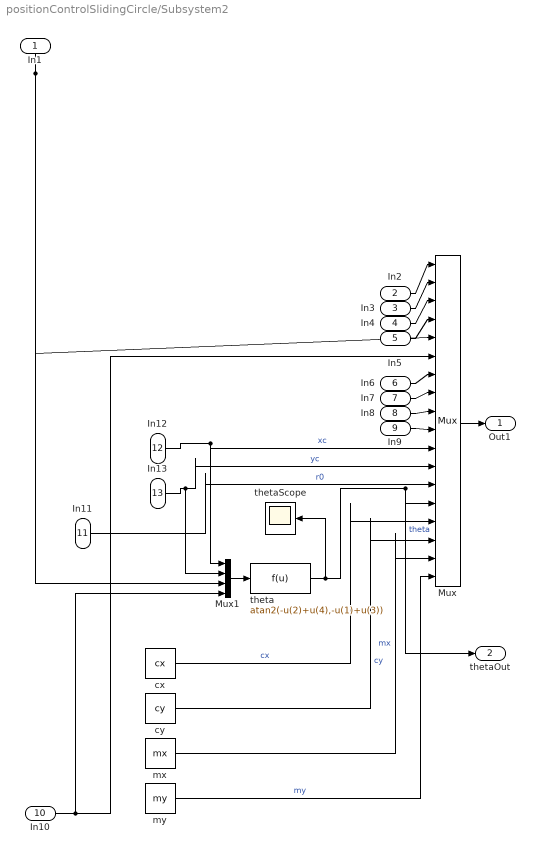
== system positionControlSlidingCircle/Subsystem2 ==
  In1 : Inport
  In2 : Inport  Port=2
  In3 : Inport  Port=3
  In4 : Inport  Port=4
  In5 : Inport  Port=5
  In6 : Inport  Port=6
  In7 : Inport  Port=7
  In8 : Inport  Port=8
  In9 : Inport  Port=9
  In10 : Inport  Port=10
  In11 : Inport  Port=11
  In12 : Inport  Port=12
  In13 : Inport  Port=13
  Mux : Mux  Inputs=18
  Mux1 : Mux
  cx : Constant  Value=cx  OutDataType=fixdt(1, 16)  OutScaling=2^0
  cy : Constant  Value=cy  OutDataType=fixdt(1, 16)  OutScaling=2^0
  mx : Constant  Value=mx  OutDataType=fixdt(1, 16)  OutScaling=2^0
  my : Constant  Value=my  OutDataType=fixdt(1, 16)  OutScaling=2^0
  theta : Fcn  Expr=atan2(-u(2)+u(4),-u(1)+u(3))
  thetaScope : Scope
      settings: SaveName=ScopeData2
  Out1 : Outport
  thetaOut : Outport  Port=2
  wires:
  theta/1 -> thetaScope/1, Mux/14, thetaOut/1  "theta"
  Mux1/1 -> theta/1
  my/1 -> Mux/18  "my"
  mx/1 -> Mux/17  "mx"
  cy/1 -> Mux/16  "cy"
  cx/1 -> Mux/15  "cx"
  In11/1 -> Mux/13  "r0"
  In13/1 -> Mux/12, Mux1/2  "yc"
  In12/1 -> Mux/11, Mux1/1  "xc"
  In10/1 -> Mux1/4, Mux/6
  In1/1 -> Mux1/3, Mux/5
  In2/1 -> Mux/1
  In3/1 -> Mux/2
  In4/1 -> Mux/3
  In5/1 -> Mux/4
  In6/1 -> Mux/7
  In7/1 -> Mux/8
  In8/1 -> Mux/9
  Mux/1 -> Out1/1
  In9/1 -> Mux/10

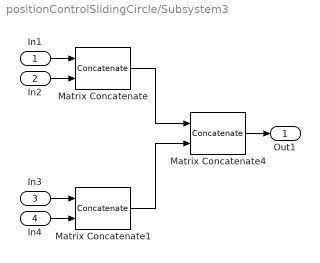
== system positionControlSlidingCircle/Subsystem3 ==
  In1 : Inport
  In2 : Inport  Port=2
  In3 : Inport  Port=3
  In4 : Inport  Port=4
  Matrix Concatenate : Concatenate  Mode=Vector  ConcatenateDimension=2
  Matrix Concatenate1 : Concatenate  Mode=Vector  ConcatenateDimension=2
  Matrix Concatenate4 : Concatenate  Mode=Multidimensional array  ConcatenateDimension=2
  Out1 : Outport
  wires:
  Matrix Concatenate/1 -> Matrix Concatenate4/1
  Matrix Concatenate1/1 -> Matrix Concatenate4/2
  In1/1 -> Matrix Concatenate/1
  In2/1 -> Matrix Concatenate/2
  Matrix Concatenate4/1 -> Out1/1
  In3/1 -> Matrix Concatenate1/1
  In4/1 -> Matrix Concatenate1/2

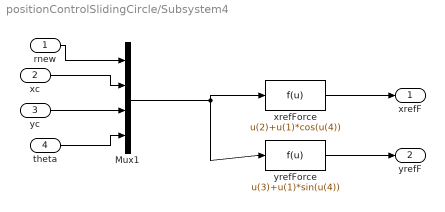
== system positionControlSlidingCircle/Subsystem4 ==
  rnew : Inport
  xc : Inport  Port=2
  yc : Inport  Port=3
  theta : Inport  Port=4
  Mux1 : Mux
  xrefForce : Fcn  Expr=u(2)+u(1)*cos(u(4))
  yrefForce : Fcn  Expr=u(3)+u(1)*sin(u(4))
  xrefF : Outport  OutDataType=fixdt(1, 16)  OutScaling=2^0
  yrefF : Outport  Port=2  OutDataType=fixdt(1, 16)  OutScaling=2^0
  wires:
  xc/1 -> Mux1/2
  yc/1 -> Mux1/3
  rnew/1 -> Mux1/1
  Mux1/1 -> xrefForce/1, yrefForce/1
  theta/1 -> Mux1/4
  xrefForce/1 -> xrefF/1
  yrefForce/1 -> yrefF/1

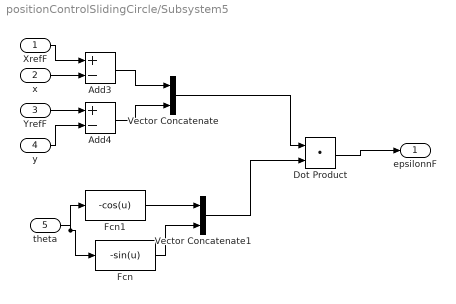
== system positionControlSlidingCircle/Subsystem5 ==
  XrefF : Inport
  x : Inport  Port=2
  YrefF : Inport  Port=3
  y : Inport  Port=4
  theta : Inport  Port=5
  Add3 : Sum  Inputs=+-  OutDataType=fixdt(1, 16)  OutScaling=2^-10
  Add4 : Sum  Inputs=+-  OutDataType=fixdt(1, 16)  OutScaling=2^-10
  Dot Product : DotProduct  OutDataType=fixdt(1, 16)  OutScaling=2^-10  InputSameDT=on  OutDataTypeStr=Inherit: Inherit via internal rule
  Fcn : Fcn  Expr=-sin(u)
  Fcn1 : Fcn  Expr=-cos(u)
  Vector Concatenate : Concatenate  Mode=Vector
  Vector Concatenate1 : Concatenate  Mode=Vector
  epsilonnF : Outport  OutDataType=fixdt(1, 16)  OutScaling=2^0
  wires:
  Add3/1 -> Vector Concatenate/1
  Add4/1 -> Vector Concatenate/2
  x/1 -> Add3/2
  y/1 -> Add4/2
  XrefF/1 -> Add3/1
  Vector Concatenate/1 -> Dot Product/1
  YrefF/1 -> Add4/1
  theta/1 -> Fcn1/1, Fcn/1
  Fcn1/1 -> Vector Concatenate1/1
  Fcn/1 -> Vector Concatenate1/2
  Vector Concatenate1/1 -> Dot Product/2
  Dot Product/1 -> epsilonnF/1

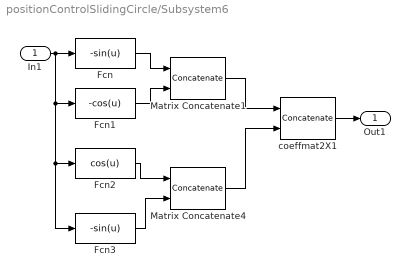
== system positionControlSlidingCircle/Subsystem6 ==
  In1 : Inport
  Fcn : Fcn  Expr=-sin(u)
  Fcn1 : Fcn  Expr=-cos(u)
  Fcn2 : Fcn  Expr=cos(u)
  Fcn3 : Fcn  Expr=-sin(u)
  Matrix Concatenate1 : Concatenate  Mode=Multidimensional array  ConcatenateDimension=2
  Matrix Concatenate4 : Concatenate  Mode=Multidimensional array  ConcatenateDimension=2
  coeffmat2X1 : Concatenate  Mode=Multidimensional array
  Out1 : Outport
  wires:
  Matrix Concatenate1/1 -> coeffmat2X1/1
  Matrix Concatenate4/1 -> coeffmat2X1/2
  Fcn/1 -> Matrix Concatenate1/1
  Fcn1/1 -> Matrix Concatenate1/2
  Fcn2/1 -> Matrix Concatenate4/1
  Fcn3/1 -> Matrix Concatenate4/2
  In1/1 -> Fcn/1, Fcn1/1, Fcn2/1, Fcn3/1
  coeffmat2X1/1 -> Out1/1

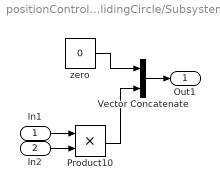
== system positionControlSlidingCircle/Subsystem7 ==
  In1 : Inport
  In2 : Inport  Port=2
  Product10 : Product  OutDataType=fixdt(1, 16)  OutScaling=2^0  RndMeth=Zero
  Vector Concatenate : Concatenate  Mode=Vector
  zero : Constant  Value=0  OutDataType=fixdt(1, 16)  OutScaling=2^0
  Out1 : Outport
  wires:
  zero/1 -> Vector Concatenate/1
  Product10/1 -> Vector Concatenate/2
  Vector Concatenate/1 -> Out1/1
  In1/1 -> Product10/1
  In2/1 -> Product10/2

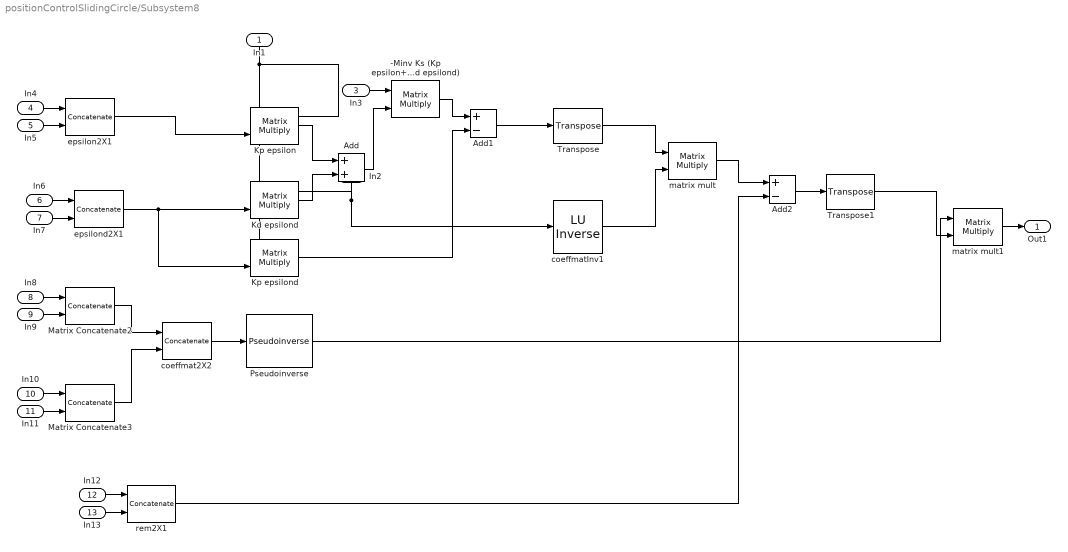
== system positionControlSlidingCircle/Subsystem8 ==
  In1 : Inport
  In2 : Inport  Port=2
  In3 : Inport  Port=3
  In4 : Inport  Port=4
  In5 : Inport  Port=5
  In6 : Inport  Port=6
  In7 : Inport  Port=7
  In8 : Inport  Port=8
  In9 : Inport  Port=9
  In10 : Inport  Port=10
  In11 : Inport  Port=11
  In12 : Inport  Port=12
  In13 : Inport  Port=13
  -Minv Ks (Kp epsilon+Kd epsilond) : Product  Multiplication=Matrix(*)  OutDataType=sfix(16)  OutScaling=2^0
  Add : Sum  OutDataType=fixdt(1, 16)  OutScaling=2^-10
  Add1 : Sum  Inputs=+-  OutDataType=fixdt(1, 16)  OutScaling=2^-10
  Add2 : Sum  Inputs=+-  OutDataType=fixdt(1, 16)  OutScaling=2^-10
  Kd epsilond : Product  Multiplication=Matrix(*)  OutDataType=sfix(16)  OutScaling=2^0
  Kp epsilon : Product  Multiplication=Matrix(*)  OutDataType=sfix(16)  OutScaling=2^0
  Kp epsilond : Product  Multiplication=Matrix(*)  OutDataType=sfix(16)  OutScaling=2^0
  Matrix Concatenate2 : Concatenate  Mode=Multidimensional array  ConcatenateDimension=2
  Matrix Concatenate3 : Concatenate  Mode=Multidimensional array  ConcatenateDimension=2
  Pseudoinverse : dspinverses/Pseudoinverse  wanterr=off
  Transpose : dspmtrx3/Transpose  SystemSampleTime=-1  Hermitian=off  overflowFlag=off
  Transpose1 : dspmtrx3/Transpose  SystemSampleTime=-1  Hermitian=off  overflowFlag=off
  coeffmat2X2 : Concatenate  Mode=Multidimensional array
  coeffmatInv1 : dspinverses/ LU Inverse  SystemSampleTime=-1
  epsilon2X1 : Concatenate  Mode=Vector  ConcatenateDimension=2
  epsilond2X1 : Concatenate  Mode=Vector  ConcatenateDimension=2
  matrix mult : Product  Multiplication=Matrix(*)  OutDataType=sfix(16)  OutScaling=2^0
  matrix mult1 : Product  Multiplication=Matrix(*)  OutDataType=sfix(16)  OutScaling=2^0
  rem2X1 : Concatenate  Mode=Vector  ConcatenateDimension=2
  Out1 : Outport
  wires:
  Transpose1/1 -> matrix mult1/2
  Add2/1 -> Transpose1/1
  Transpose/1 -> matrix mult/1
  Pseudoinverse/1 -> matrix mult1/1
  rem2X1/1 -> Add2/2
  matrix mult/1 -> Add2/1
  coeffmatInv1/1 -> matrix mult/2
  Add1/1 -> Transpose/1
  Kp epsilond/1 -> Add1/2
  -Minv Ks (Kp epsilon+Kd epsilond)/1 -> Add1/1
  Add/1 -> -Minv Ks (Kp epsilon+Kd epsilond)/2
  Kd epsilond/1 -> Add/2
  Kp epsilon/1 -> Add/1
  epsilond2X1/1 -> Kd epsilond/2, Kp epsilond/2
  In2/1 -> coeffmatInv1/1, Kd epsilond/1
  epsilon2X1/1 -> Kp epsilon/2
  In1/1 -> Kp epsilond/1, Kp epsilon/1
  coeffmat2X2/1 -> Pseudoinverse/1
  Matrix Concatenate3/1 -> coeffmat2X2/2
  Matrix Concatenate2/1 -> coeffmat2X2/1
  In3/1 -> -Minv Ks (Kp epsilon+Kd epsilond)/1
  In4/1 -> epsilon2X1/1
  In5/1 -> epsilon2X1/2
  In6/1 -> epsilond2X1/1
  In7/1 -> epsilond2X1/2
  matrix mult1/1 -> Out1/1
  In8/1 -> Matrix Concatenate2/1
  In9/1 -> Matrix Concatenate2/2
  In10/1 -> Matrix Concatenate3/1
  In11/1 -> Matrix Concatenate3/2
  In12/1 -> rem2X1/1
  In13/1 -> rem2X1/2

== system positionControlSlidingCircle/RTI Data/RTI Data Store ==
  RTI Data Store : Subsystem
      mask Type: RTI_DATA_STORE
      mask Description:
      | RTI Data Store Block. This block is used by RTI to store internal model dependent data. Deleting this block will result in data loss.
      | 
      | NEVER DELETE, COPY, OR MODIFY THIS BLOCK!
      mask Help:
      | RTI Data Store Block. This block is used by RTI to store internal model dependent data. Deleting this block will result in data loss.
      | 
      | NEVER DELETE, COPY, OR MODIFY THIS BLOCK!
      mask Display: text(0.5, 0.5, ' ', 'HorizontalAlignment', 'center');

== system positionControlSlidingCircle/RTI Data/RTI Data Store/RTI Data Store ==
  RTI Data Store : Subsystem
      mask Type: RTI_DATA_STORE
      mask Description:
      | RTI Data Store Block. This block is used by RTI to store internal model dependent data. Deleting this block will result in data loss.
      | 
      | NEVER DELETE, COPY, OR MODIFY THIS BLOCK!
      mask Help:
      | RTI Data Store Block. This block is used by RTI to store internal model dependent data. Deleting this block will result in data loss.
      | 
      | NEVER DELETE, COPY, OR MODIFY THIS BLOCK!
      mask Display: text(0.5, 0.5, ' ', 'HorizontalAlignment', 'center');

== system positionControlSlidingCircle/RTI Data/RTI Data Store/RTI Data Store/RTI Data Store ==
  RTI Data Store : Subsystem
      mask Type: RTI_DATA_STORE
      mask Description:
      | RTI Data Store Block. This block is used by RTI to store internal model dependent data. Deleting this block will result in data loss.
      | 
      | NEVER DELETE, COPY, OR MODIFY THIS BLOCK!
      mask Help:
      | RTI Data Store Block. This block is used by RTI to store internal model dependent data. Deleting this block will result in data loss.
      | 
      | NEVER DELETE, COPY, OR MODIFY THIS BLOCK!
      mask Display: text(0.5, 0.5, ' ', 'HorizontalAlignment', 'center');

== system positionControlSlidingCircle/RTI Data/RTI Data Store/RTI Data Store/RTI Data Store/RTI Data Store ==
